simulink model "EX65c"  (R2014b)
settings: Solver=FixedStepDiscrete  StartTime=0.0  StopTime=5.24288  RelTol=1e-3
libraries: commrandsrc2 x1
settings Model: Creator=Silage  LastModifiedBy=Silage
settings DataIOCC: SignalLoggingSaveFormat=ModelDataLogs
settings OptimizationCC: ExpressionDepthLimit=2147483647
settings DebuggingCC: UnderspecifiedInitializationDetection=Classic  MergeDetectMultiDrivingBlocksExec=none  FcnCallInpInsideContextMsg=EnableAllAsWarning  StateNameClashWarn=warning
settings GRTTargetCC: CombineOutputUpdateFcns=off  GRTInterface=on

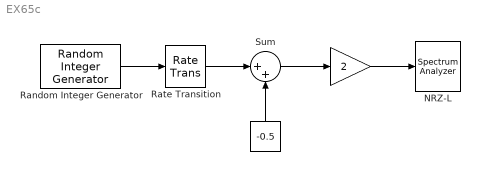
== system EX65c ==
  " " : Constant  Value=-0.5
  "   " : Gain  Gain=2
  NRZ-L : SpectrumAnalyzer
  Random Integer Generator : commrandsrc2/Random Integer Generator  mul=2  seed=randseed  Ts=1e-3  frameBased=off  sampPerFrame=1  orient=on  outDataType=double
  Rate Transition : RateTransition  OutPortSampleTime=2e-5
  Sum : Sum  Inputs=|++
  wires:
  Random Integer Generator/1 -> Rate Transition/1
  Rate Transition/1 -> Sum/1
  " "/1 -> Sum/2
  Sum/1 -> "   "/1
  "   "/1 -> NRZ-L/1
